simulink model "towTest_dualWinch"  (R2020a)
settings: Solver=FixedStepAuto  StartTime=0.0  StopTime=inf  FixedStep=Ts  RelTol=1e-3  EnableMultiTasking=on
undefined symbols (not defined in the file): encAng_trig, IO397, standard
libraries: xpcutilitieslib x52, hdlsllib x29, simulink x11, slrtlib x9, dspsigops x5, xpcseriallib x2, speedgoatlib_fpga_quadrature x2, powerlib_meascontrol x2, xpcrtudplib x2, speedgoatlib_fpga_dio x1, speedgoatlib_fpga_analog_io x1, speedgoatlib_IO581 x1
(part 2 of 2)

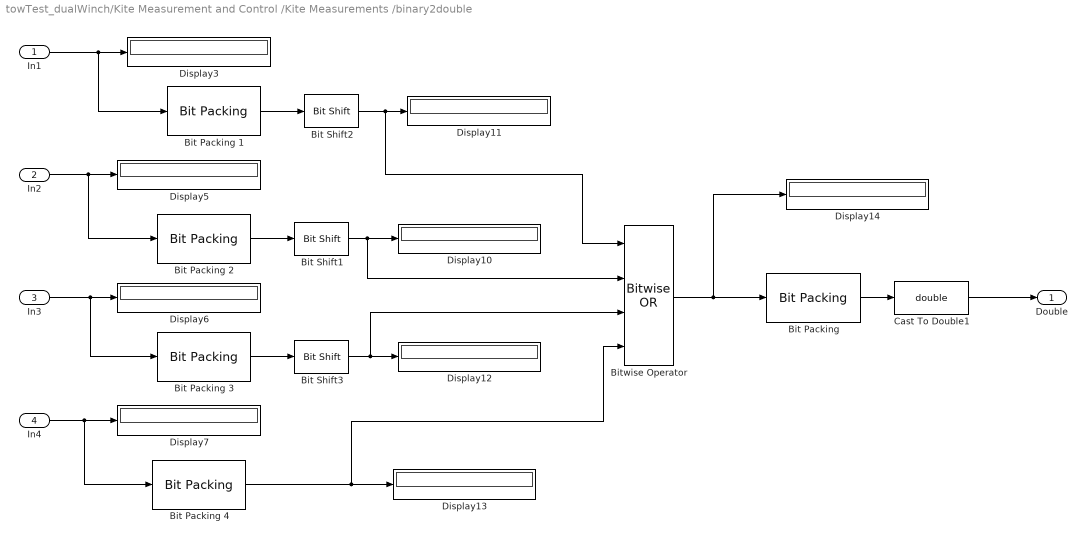
== system towTest_dualWinch/Kite Measurement and Control /Kite Measurements /binary2double ==
  In1 : Inport
  In2 : Inport  Port=2
  In3 : Inport  Port=3
  In4 : Inport  Port=4
  Bit Packing {,1..4} (5 alike) : xpcutilitieslib/Bit Packing 
      settings: SourceProductBaseCode=XP
  Bit Shift1 : hdlsllib/Logic and Bit Operations/Bit Shift  mode=Shift Left Logical  N=16
  Bit Shift2 : hdlsllib/Logic and Bit Operations/Bit Shift  mode=Shift Left Logical  N=24
  Bit Shift3 : hdlsllib/Logic and Bit Operations/Bit Shift  mode=Shift Left Logical  N=8
  Bitwise Operator : simulink/Logic and Bit Operations/Bitwise Operator  logicop=OR  UseBitMask=off  NumInputPorts=4  BitMask=bin2dec('00000000')  BitMaskRealWorld=Stored Integer
  Cast To Double1 : DataTypeConversion  OutDataTypeStr=double
  Display{3,5..7,10..14} (9 alike) : Display
      settings: Format=hex (Stored Integer)
  Double : Outport
  wires:
  Bit Shift1/1 -> Bitwise Operator/2, Display10/1
  Bitwise Operator/1 -> Display14/1, "Bit Packing "/1
  Bit Packing 1/1 -> Bit Shift2/1
  Bit Packing 4/1 -> Bitwise Operator/4, Display13/1
  In1/1 -> Bit Packing 1/1, Display3/1
  In3/1 -> Bit Packing 3/1, Display6/1
  Bit Shift2/1 -> Bitwise Operator/1, Display11/1
  Bit Packing 2/1 -> Bit Shift1/1
  "Bit Packing "/1 -> Cast To Double1/1
  Bit Shift3/1 -> Bitwise Operator/3, Display12/1
  Bit Packing 3/1 -> Bit Shift3/1
  In2/1 -> Bit Packing 2/1, Display5/1
  In4/1 -> Bit Packing 4/1, Display7/1
  Cast To Double1/1 -> Double/1

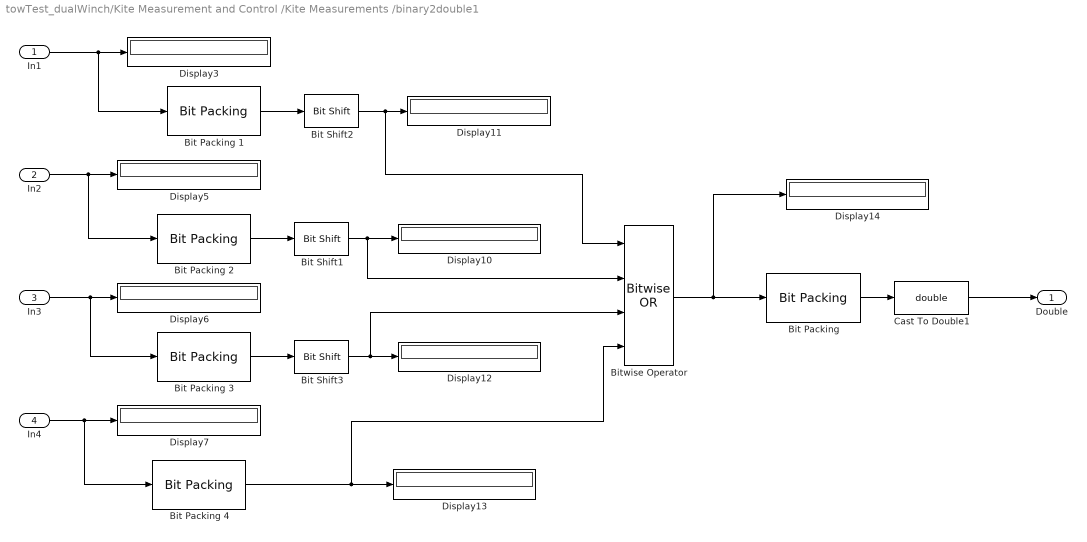
== system towTest_dualWinch/Kite Measurement and Control /Kite Measurements /binary2double1 ==
  In1 : Inport
  In2 : Inport  Port=2
  In3 : Inport  Port=3
  In4 : Inport  Port=4
  Bit Packing {,1..4} (5 alike) : xpcutilitieslib/Bit Packing 
      settings: SourceProductBaseCode=XP
  Bit Shift1 : hdlsllib/Logic and Bit Operations/Bit Shift  mode=Shift Left Logical  N=16
  Bit Shift2 : hdlsllib/Logic and Bit Operations/Bit Shift  mode=Shift Left Logical  N=24
  Bit Shift3 : hdlsllib/Logic and Bit Operations/Bit Shift  mode=Shift Left Logical  N=8
  Bitwise Operator : simulink/Logic and Bit Operations/Bitwise Operator  logicop=OR  UseBitMask=off  NumInputPorts=4  BitMask=bin2dec('00000000')  BitMaskRealWorld=Stored Integer
  Cast To Double1 : DataTypeConversion  OutDataTypeStr=double
  Display{3,5..7,10..14} (9 alike) : Display
      settings: Format=hex (Stored Integer)
  Double : Outport
  wires:
  Bit Shift1/1 -> Bitwise Operator/2, Display10/1
  Bitwise Operator/1 -> Display14/1, "Bit Packing "/1
  Bit Packing 1/1 -> Bit Shift2/1
  Bit Packing 4/1 -> Bitwise Operator/4, Display13/1
  In1/1 -> Bit Packing 1/1, Display3/1
  In3/1 -> Bit Packing 3/1, Display6/1
  Bit Shift2/1 -> Bitwise Operator/1, Display11/1
  Bit Packing 2/1 -> Bit Shift1/1
  "Bit Packing "/1 -> Cast To Double1/1
  Bit Shift3/1 -> Bitwise Operator/3, Display12/1
  Bit Packing 3/1 -> Bit Shift3/1
  In2/1 -> Bit Packing 2/1, Display5/1
  In4/1 -> Bit Packing 4/1, Display7/1
  Cast To Double1/1 -> Double/1

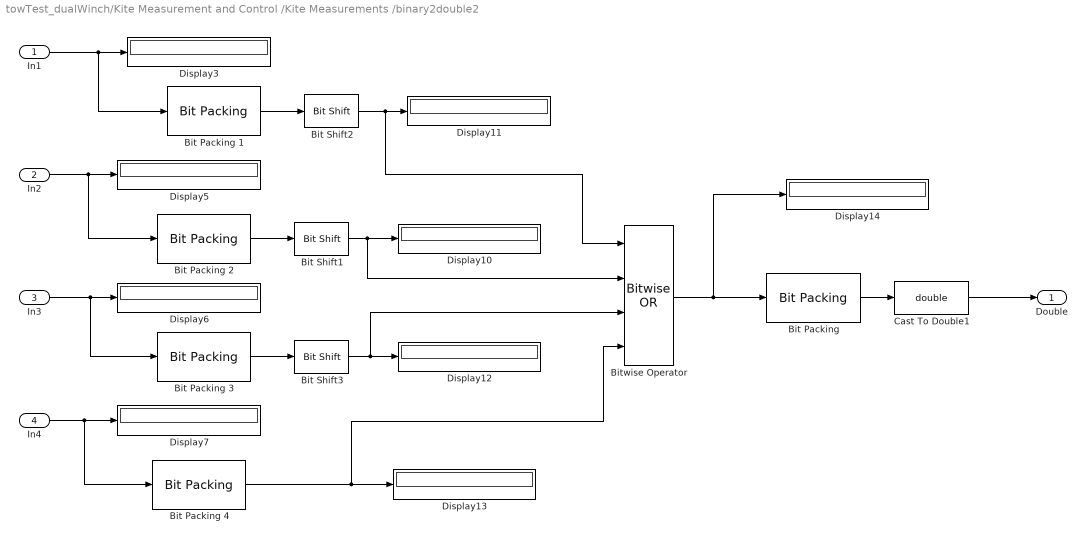
== system towTest_dualWinch/Kite Measurement and Control /Kite Measurements /binary2double2 ==
  In1 : Inport
  In2 : Inport  Port=2
  In3 : Inport  Port=3
  In4 : Inport  Port=4
  Bit Packing {,1..4} (5 alike) : xpcutilitieslib/Bit Packing 
      settings: SourceProductBaseCode=XP
  Bit Shift1 : hdlsllib/Logic and Bit Operations/Bit Shift  mode=Shift Left Logical  N=16
  Bit Shift2 : hdlsllib/Logic and Bit Operations/Bit Shift  mode=Shift Left Logical  N=24
  Bit Shift3 : hdlsllib/Logic and Bit Operations/Bit Shift  mode=Shift Left Logical  N=8
  Bitwise Operator : simulink/Logic and Bit Operations/Bitwise Operator  logicop=OR  UseBitMask=off  NumInputPorts=4  BitMask=bin2dec('00000000')  BitMaskRealWorld=Stored Integer
  Cast To Double1 : DataTypeConversion  OutDataTypeStr=double
  Display{3,5..7,10..14} (9 alike) : Display
      settings: Format=hex (Stored Integer)
  Double : Outport
  wires:
  Bit Shift1/1 -> Bitwise Operator/2, Display10/1
  Bitwise Operator/1 -> Display14/1, "Bit Packing "/1
  Bit Packing 1/1 -> Bit Shift2/1
  Bit Packing 4/1 -> Bitwise Operator/4, Display13/1
  In1/1 -> Bit Packing 1/1, Display3/1
  In3/1 -> Bit Packing 3/1, Display6/1
  Bit Shift2/1 -> Bitwise Operator/1, Display11/1
  Bit Packing 2/1 -> Bit Shift1/1
  "Bit Packing "/1 -> Cast To Double1/1
  Bit Shift3/1 -> Bitwise Operator/3, Display12/1
  Bit Packing 3/1 -> Bit Shift3/1
  In2/1 -> Bit Packing 2/1, Display5/1
  In4/1 -> Bit Packing 4/1, Display7/1
  Cast To Double1/1 -> Double/1

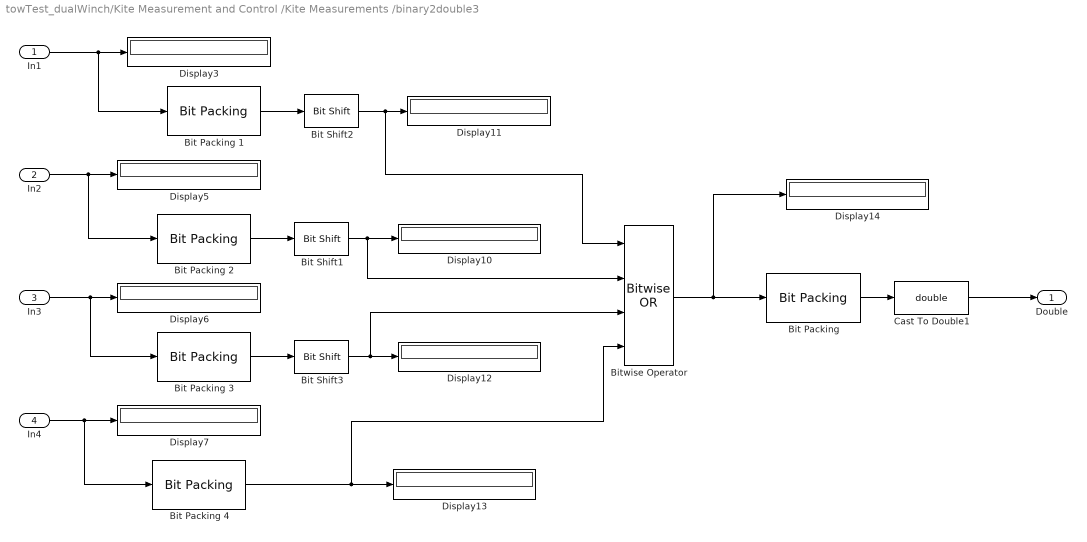
== system towTest_dualWinch/Kite Measurement and Control /Kite Measurements /binary2double3 ==
  In1 : Inport
  In2 : Inport  Port=2
  In3 : Inport  Port=3
  In4 : Inport  Port=4
  Bit Packing {,1..4} (5 alike) : xpcutilitieslib/Bit Packing 
      settings: SourceProductBaseCode=XP
  Bit Shift1 : hdlsllib/Logic and Bit Operations/Bit Shift  mode=Shift Left Logical  N=16
  Bit Shift2 : hdlsllib/Logic and Bit Operations/Bit Shift  mode=Shift Left Logical  N=24
  Bit Shift3 : hdlsllib/Logic and Bit Operations/Bit Shift  mode=Shift Left Logical  N=8
  Bitwise Operator : simulink/Logic and Bit Operations/Bitwise Operator  logicop=OR  UseBitMask=off  NumInputPorts=4  BitMask=bin2dec('00000000')  BitMaskRealWorld=Stored Integer
  Cast To Double1 : DataTypeConversion  OutDataTypeStr=double
  Display{3,5..7,10..14} (9 alike) : Display
      settings: Format=hex (Stored Integer)
  Double : Outport
  wires:
  Bit Shift1/1 -> Bitwise Operator/2, Display10/1
  Bitwise Operator/1 -> Display14/1, "Bit Packing "/1
  Bit Packing 1/1 -> Bit Shift2/1
  Bit Packing 4/1 -> Bitwise Operator/4, Display13/1
  In1/1 -> Bit Packing 1/1, Display3/1
  In3/1 -> Bit Packing 3/1, Display6/1
  Bit Shift2/1 -> Bitwise Operator/1, Display11/1
  Bit Packing 2/1 -> Bit Shift1/1
  "Bit Packing "/1 -> Cast To Double1/1
  Bit Shift3/1 -> Bitwise Operator/3, Display12/1
  Bit Packing 3/1 -> Bit Shift3/1
  In2/1 -> Bit Packing 2/1, Display5/1
  In4/1 -> Bit Packing 4/1, Display7/1
  Cast To Double1/1 -> Double/1

== system towTest_dualWinch/Kite Measurement and Control /Kite Measurements /binary2double4 ==
  In1 : Inport
  In2 : Inport  Port=2
  In3 : Inport  Port=3
  In4 : Inport  Port=4
  Bit Packing {,1..4} (5 alike) : xpcutilitieslib/Bit Packing 
      settings: SourceProductBaseCode=XP
  Bit Shift1 : hdlsllib/Logic and Bit Operations/Bit Shift  mode=Shift Left Logical  N=16
  Bit Shift2 : hdlsllib/Logic and Bit Operations/Bit Shift  mode=Shift Left Logical  N=24
  Bit Shift3 : hdlsllib/Logic and Bit Operations/Bit Shift  mode=Shift Left Logical  N=8
  Bitwise Operator : simulink/Logic and Bit Operations/Bitwise Operator  logicop=OR  UseBitMask=off  NumInputPorts=4  BitMask=bin2dec('00000000')  BitMaskRealWorld=Stored Integer
  Cast To Double1 : DataTypeConversion  OutDataTypeStr=double
  Display{3,5..7,10..14} (9 alike) : Display
      settings: Format=hex (Stored Integer)
  Double : Outport
  wires:
  Bit Shift1/1 -> Bitwise Operator/2, Display10/1
  Bitwise Operator/1 -> Display14/1, "Bit Packing "/1
  Bit Packing 1/1 -> Bit Shift2/1
  Bit Packing 4/1 -> Bitwise Operator/4, Display13/1
  In1/1 -> Bit Packing 1/1, Display3/1
  In3/1 -> Bit Packing 3/1, Display6/1
  Bit Shift2/1 -> Bitwise Operator/1, Display11/1
  Bit Packing 2/1 -> Bit Shift1/1
  "Bit Packing "/1 -> Cast To Double1/1
  Bit Shift3/1 -> Bitwise Operator/3, Display12/1
  Bit Packing 3/1 -> Bit Shift3/1
  In2/1 -> Bit Packing 2/1, Display5/1
  In4/1 -> Bit Packing 4/1, Display7/1
  Cast To Double1/1 -> Double/1

== system towTest_dualWinch/Kite Measurement and Control /Kite Measurements /binary2double5 ==
  In1 : Inport
  In2 : Inport  Port=2
  In3 : Inport  Port=3
  In4 : Inport  Port=4
  Bit Packing {,1..4} (5 alike) : xpcutilitieslib/Bit Packing 
      settings: SourceProductBaseCode=XP
  Bit Shift1 : hdlsllib/Logic and Bit Operations/Bit Shift  mode=Shift Left Logical  N=16
  Bit Shift2 : hdlsllib/Logic and Bit Operations/Bit Shift  mode=Shift Left Logical  N=24
  Bit Shift3 : hdlsllib/Logic and Bit Operations/Bit Shift  mode=Shift Left Logical  N=8
  Bitwise Operator : simulink/Logic and Bit Operations/Bitwise Operator  logicop=OR  UseBitMask=off  NumInputPorts=4  BitMask=bin2dec('00000000')  BitMaskRealWorld=Stored Integer
  Cast To Double1 : DataTypeConversion  OutDataTypeStr=double
  Display{3,5..7,10..14} (9 alike) : Display
      settings: Format=hex (Stored Integer)
  Double : Outport
  wires:
  Bit Shift1/1 -> Bitwise Operator/2, Display10/1
  Bitwise Operator/1 -> Display14/1, "Bit Packing "/1
  Bit Packing 1/1 -> Bit Shift2/1
  Bit Packing 4/1 -> Bitwise Operator/4, Display13/1
  In1/1 -> Bit Packing 1/1, Display3/1
  In3/1 -> Bit Packing 3/1, Display6/1
  Bit Shift2/1 -> Bitwise Operator/1, Display11/1
  Bit Packing 2/1 -> Bit Shift1/1
  "Bit Packing "/1 -> Cast To Double1/1
  Bit Shift3/1 -> Bitwise Operator/3, Display12/1
  Bit Packing 3/1 -> Bit Shift3/1
  In2/1 -> Bit Packing 2/1, Display5/1
  In4/1 -> Bit Packing 4/1, Display7/1
  Cast To Double1/1 -> Double/1

== system towTest_dualWinch/Kite Measurement and Control /Kite Measurements /binary2double6 ==
  In1 : Inport
  In2 : Inport  Port=2
  In3 : Inport  Port=3
  In4 : Inport  Port=4
  Bit Packing {,1..4} (5 alike) : xpcutilitieslib/Bit Packing 
      settings: SourceProductBaseCode=XP
  Bit Shift1 : hdlsllib/Logic and Bit Operations/Bit Shift  mode=Shift Left Logical  N=16
  Bit Shift2 : hdlsllib/Logic and Bit Operations/Bit Shift  mode=Shift Left Logical  N=24
  Bit Shift3 : hdlsllib/Logic and Bit Operations/Bit Shift  mode=Shift Left Logical  N=8
  Bitwise Operator : simulink/Logic and Bit Operations/Bitwise Operator  logicop=OR  UseBitMask=off  NumInputPorts=4  BitMask=bin2dec('00000000')  BitMaskRealWorld=Stored Integer
  Cast To Double1 : DataTypeConversion  OutDataTypeStr=double
  Display{3,5..7,10..14} (9 alike) : Display
      settings: Format=hex (Stored Integer)
  Double : Outport
  wires:
  Bit Shift1/1 -> Bitwise Operator/2, Display10/1
  Bitwise Operator/1 -> Display14/1, "Bit Packing "/1
  Bit Packing 1/1 -> Bit Shift2/1
  Bit Packing 4/1 -> Bitwise Operator/4, Display13/1
  In1/1 -> Bit Packing 1/1, Display3/1
  In3/1 -> Bit Packing 3/1, Display6/1
  Bit Shift2/1 -> Bitwise Operator/1, Display11/1
  Bit Packing 2/1 -> Bit Shift1/1
  "Bit Packing "/1 -> Cast To Double1/1
  Bit Shift3/1 -> Bitwise Operator/3, Display12/1
  Bit Packing 3/1 -> Bit Shift3/1
  In2/1 -> Bit Packing 2/1, Display5/1
  In4/1 -> Bit Packing 4/1, Display7/1
  Cast To Double1/1 -> Double/1

== matlab function towTest_dualWinch/LAS_Calculation/ifOutsideBounds ==
  data: u input; y output
function y = fcn(u)

if u > 180
    u = u - 360;
elseif u < -180
    u = u + 360;    
end

y = u;

== matlab function towTest_dualWinch/LAS_Calculation/LAS Measurement Corrections ==
  data: elev output; elev_encoder input; azi output; azi_encoder input
function [elev,azi] = fcn(elev_encoder, azi_encoder)

% Roller radius
rollRad = 0.0381;   % m

% Elevation joint, azimuth hub
elLink.a = 0.0229997;   % m
elLink.alpha = -pi/2;   % rad
elLink.d = 0;
elLink.theta = -elev_encoder; % Elevation encoder (change to pipe in data)

% Azimuth joint, boom
azLink.a = 0.49424;  % m
azLink.alpha = 0;
azLink.d = 0.0304;   % m
azLink.theta = azi_encoder; % Azimuth encoder (change to pipe in data)

% Elevation joint to end effector
Ael = jointTform(elLink);
Aaz = jointTform(azLink);
T = Ael*Aaz; % Transformation matrix

% Information above will be used in dynamics calculations
% --------------------------------------------------------------
% Information below is used for correcting tether angle
% Assume that the tether is tangent to the roller

endEffCart = T(1:3,4); % Enf effector Cartesian coordinates

% Roller center to end effector
hubCart = [-0.0717;-0.06785;0]; % Roller center to elevation joint
rc2ef = hubCart + endEffCart;

% Magnitude of roll center to end effector (2D)
rc2ef_Hyp = sqrt(rc2ef(1)^2 + rc2ef(2)^2);

% Elevation angle between end eff. to center and end eff. to surface
thetaOppHyp = asin(rollRad/rc2ef_Hyp);

% Elevation angle between end eff. to center and horizontal
thetaElevation = asin(-rc2ef(2)/rc2ef_Hyp);

% Angle from vertical to tether contact point on the roller
rollAng = thetaElevation-thetaOppHyp;

% Vector approximation from roller center to contact surface
% Map roller contact angle to elevation angle
rc2rsApprox = [cos(elLink.theta) -sin(elLink.theta) 0;
              sin(elLink.theta) cos(elLink.theta)   0;
              0                 0                   1]*[0;-rollRad;0];

% Vector from roller center to contact surface
% Using center-surface angle determined by trig
rc2rs = [cos(-rollAng) -sin(-rollAng) 0;
        sin(-rollAng)  cos(-rollAng)  0;
        0              0              1]*[0;-rollRad;0];

% Vector from contact surface to end effector (APPROXIMATION)
tetherVecApprox = rc2ef - rc2rsApprox;

% Vector from contact surface to end effector (FINAL)
tetherVec = rc2ef - rc2rs;

%% Block output

% Change block output spherical
    elev = asin(-tetherVecApprox(2)/norm(tetherVecApprox));
    azi = asin(-tetherVecApprox(3)/norm(tetherVecApprox)/cos(elev));

end

function A = jointTform(link)

% Transforms from the end effector to the base frame in the order: joint
% angle, then link offset, then link 

% INPUT %
% link.theta - joint angle (radians)
% link.d     - link offset
% link.a     - link length
% linkalpha - link twist (radians)

% OUTPUT %
% A - homogeneous transform matrix

At = [cos(link.theta) -sin(link.theta) 0 0;...
      sin(link.theta) cos(link.theta) 0 0;...
      0 0 1 0; 0 0 0 1];
  
Ad = [1 0 0 0; 0 1 0 0; 0 0 1 link.d; 0 0 0 1];

Aa = [1 0 0 link.a; 0 1 0 0; 0 0 1 0; 0 0 0 1];

Al = [1 0 0 0; 0 cos(link.alpha) -sin(link.alpha) 0;
      0 sin(link.alpha) cos(link.alpha) 0; 0 0 0 1];
  
A = At*Ad*Aa*Al;
end

== matlab function towTest_dualWinch/LAS_Calculation/ifOutsideBounds1 ==
  data: u input; y output
function y = fcn(u)

if u > 180
    u = u - 360;
elseif u < -180
    u = u + 360;    
end

y = u;
